simulink model "AutogiroModel"  (R2025b)
settings: Solver=FixedStepAuto  StartTime=0.0  StopTime=170  FixedStep=0.01  MaxStep=0.001  RelTol=1e-2
PreLoadFcn:
  | state = "path";
  | visual3D = true;
  | lookDistance = 500;
  | kappa = 0.1;
  | hRef = 20;
  | VRef = 30;
  | WP(:,1) = [0  0  -20]';
  | WP(:,2) = [1500  0  -20]';
  | WP(:,3) = [1500  1000 -20]';
  | WP(:,4) = [0  1000  -20]';
  | WP(:,5) = [0  0  -20]';
model workspace (MAT data in the model file):
  L1 = 3.13
undefined symbols (not defined in the file): gravity, m, rad, rho, s, WP
libraries: slpidlib x9, aerolibconvert2 x5, simulink x3, simulink_extras x3, matrix_library x2, aerolibsim3d x2, aerolibatmos2 x1, aerolibobsolete x1, aerolibasang x1, sim3dlib x1
(part 3 of 4)

== system AutogiroModel/Environment ==
  states : Inport
  Bus Creator : BusCreator  Inputs=gravity,rho
  Bus Selector : BusSelector  OutputSignals=Xe
  COESA Atmosphere Model : aerolibatmos2/COESA Atmosphere Model  units=Metric (MKS)  spec=1976 COESA-extended U.S. Standard Atmosphere  model=Profile  profile_var=High temperature  profile_percent=1%  profile_alt=5 km (16404 ft)  envelope_var=High temperature  envelope_percent=1%  action=None
  Gain : Gain  Gain=-1
  Selector : Selector  InputPortWidth=3  IndexOptions=Index vector (dialog)  Indices=[3]  OutputSizes=1
  Terminator : Terminator
  Terminator1 : Terminator
  Terminator2 : Terminator
  gravityNED : Constant  Value=[0 0 9.81]
  statesEnv : Outport
  wires:
  Gain/1 -> COESA Atmosphere Model/1
  COESA Atmosphere Model/4 -> Bus Creator/2  "rho"
  COESA Atmosphere Model/1 -> Terminator/1
  COESA Atmosphere Model/3 -> Terminator2/1
  COESA Atmosphere Model/2 -> Terminator1/1
  gravityNED/1 -> Bus Creator/1  "gravity"
  Bus Creator/1 -> statesEnv/1
  states/1 -> Bus Selector/1
  Bus Selector/1 -> Selector/1  "<Xe>"
  Selector/1 -> Gain/1

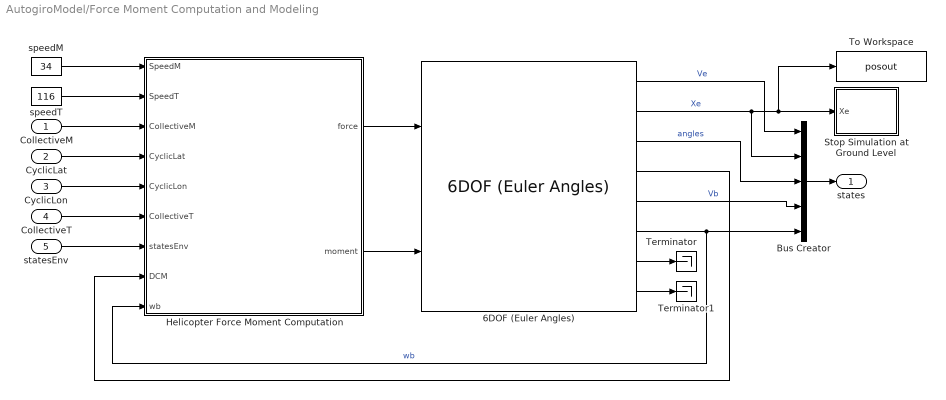
== system AutogiroModel/Force Moment Computation and Modeling ==
  CollectiveM : Inport
  CyclicLat : Inport  Port=2
  CyclicLon : Inport  Port=3
  CollectiveT : Inport  Port=4
  statesEnv : Inport  Port=5
  6DOF (Euler Angles) : aerolibobsolete/6DOF (Euler Angles)  units=Metric (MKS)  mtype=Fixed  rep=Euler Angles  xme_0=[0 0 0]  Vm_0=[0 0 0]  eul_0=[0 0 0]  pm_0=[0 0 0]  mass_0=2800  mass_e=0.5  mass_f=2.0  inertia=[3795 0 2006;0 17259 0;0 0 14639]  inertia_e=eye(3)  inertia_f=2*eye(3)  k_quat=1.0  vre_flag=on  abi_flag=off  aMode=0  xme_statename=''  Vm_statename=''  eul_statename=''  quat_statename=''  pm_statename=''  mass_statename=''
  Bus Creator : BusCreator  Inputs=5
  Helicopter Force Moment Computation : Subsystem
  Stop Simulation at Ground Level : Subsystem
  Terminator : Terminator
  Terminator1 : Terminator
  To Workspace : ToWorkspace  VariableName=posout  SaveFormat=Timeseries  SampleTime=-1
  speedM : Constant  Value=34
  speedT : Constant  Value=116
  states : Outport
  wires:
  6DOF (Euler Angles)/6 -> Bus Creator/5, Helicopter Force Moment Computation/9(wb)  "wb"
  6DOF (Euler Angles)/7 -> Terminator/1
  CyclicLat/1 -> Helicopter Force Moment Computation/4(CyclicLat)
  6DOF (Euler Angles)/5 -> Bus Creator/4  "Vb"
  6DOF (Euler Angles)/8 -> Terminator1/1
  Helicopter Force Moment Computation/1(force) -> 6DOF (Euler Angles)/1
  6DOF (Euler Angles)/2 -> To Workspace/1, Stop Simulation at Ground Level/1(Xe), Bus Creator/2  "Xe"
  6DOF (Euler Angles)/3 -> Bus Creator/3  "angles"
  CyclicLon/1 -> Helicopter Force Moment Computation/5(CyclicLon)
  CollectiveM/1 -> Helicopter Force Moment Computation/3(CollectiveM)
  CollectiveT/1 -> Helicopter Force Moment Computation/6(CollectiveT)
  Helicopter Force Moment Computation/2(moment) -> 6DOF (Euler Angles)/2
  6DOF (Euler Angles)/4 -> Helicopter Force Moment Computation/8(DCM)
  6DOF (Euler Angles)/1 -> Bus Creator/1  "Ve"
  Bus Creator/1 -> states/1
  speedM/1 -> Helicopter Force Moment Computation/1(SpeedM)
  speedT/1 -> Helicopter Force Moment Computation/2(SpeedT)
  statesEnv/1 -> Helicopter Force Moment Computation/7(statesEnv)

== system AutogiroModel/Instrument Panel ==
  Airspeed Indicator : AirspeedIndicatorBlock  LabelPosition=Hide  ScaleMin=0  ScaleMax=450
  Altimeter : AltimeterBlock  LabelPosition=Hide
  Artificial Horizon : ArtificialHorizonBlock  LabelPosition=Hide
  Climb Rate Indicator : ClimbIndicatorBlock  LabelPosition=Hide  ScaleMax=16000
  Heading Indicator : HeadingIndicatorBlock  LabelPosition=Hide
  Turn Coordinator : TurnCoordinatorBlock  LabelPosition=Hide

== system AutogiroModel/Sensor ==
  states : Inport
  Bias : Bias  Bias=0.0  SaturateOnIntegerOverflow=off
  Bus Creator : BusCreator  Inputs=5
  Bus Selector : BusSelector  OutputSignals=Ve,Xe,angles,Vb,wb
  Demux : Demux  Outputs=5
  For Each Subsystem : Subsystem  TreatAsAtomicUnit=on
  Gain : Gain  Gain=0.01
  Sum{,1..4} (5 alike) : Sum  Inputs=|++
  Uniform Random Number : UniformRandomNumber  Minimum=-0.05  Maximum=0.05  Seed=1:15  SampleTime=0.1  VectorParams1D=off
  output : Outport
  wires:
  states/1 -> Bus Selector/1
  Bus Selector/1 -> Sum/1  "<Ve>"
  Sum/1 -> Bus Creator/1  "Ve"
  Bus Creator/1 -> output/1
  Bus Selector/5 -> Sum4/1  "<wb>"
  Bus Selector/4 -> Sum3/1  "<Vb>"
  Bus Selector/3 -> Sum2/1  "<angles>"
  Bus Selector/2 -> Sum1/1  "<Xe>"
  Sum1/1 -> Bus Creator/2  "Xe"
  Sum3/1 -> Bus Creator/4  "Vb"
  Sum4/1 -> Bus Creator/5  "wb"
  Sum2/1 -> Bus Creator/3  "angles"
  Uniform Random Number/1 -> Gain/1
  Gain/1 -> Bias/1
  Bias/1 -> For Each Subsystem/1(discrete)
  Demux/1 -> Sum4/2
  Demux/2 -> Sum3/2
  Demux/3 -> Sum2/2
  Demux/4 -> Sum1/2
  Demux/5 -> Sum/2
  For Each Subsystem/1(cont) -> Demux/1

== system AutogiroModel/Visualization ==
  states : Inport
  Extract Flight Instruments : Subsystem
  Terminator{,1..5} (6 alike) : Terminator
  Variant Subsystem : Subsystem  Variant=on
  wires:
  states/1 -> Extract Flight Instruments/1(states), Variant Subsystem/1(states)
  Extract Flight Instruments/6("Turn, SlipSkid (deg)") -> Terminator5/1
  Extract Flight Instruments/5(Heading (deg)) -> Terminator4/1
  Extract Flight Instruments/4(Climb Rate (ft/min)) -> Terminator3/1
  Extract Flight Instruments/3("Roll, Pitch (deg)") -> Terminator2/1
  Extract Flight Instruments/2(Height (ft)) -> Terminator1/1
  Extract Flight Instruments/1(Airspeed (kts)) -> Terminator/1

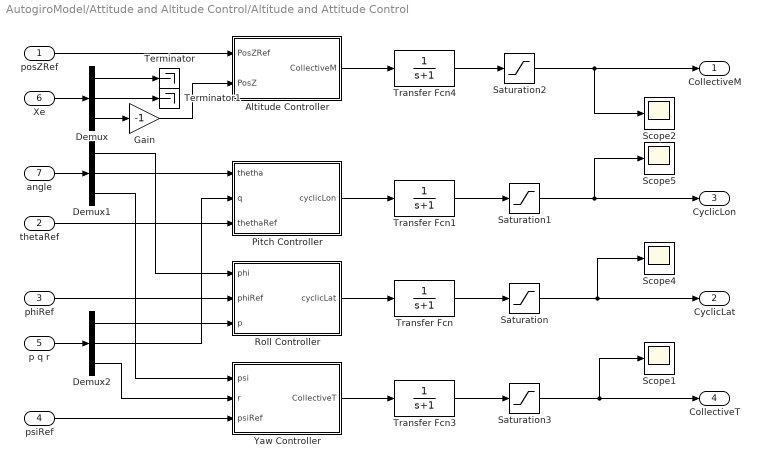
== system AutogiroModel/Attitude and Altitude Control/Altitude and Attitude Control ==
  posZRef : Inport
  thetaRef : Inport  Port=2
  phiRef : Inport  Port=3
  psiRef : Inport  Port=4
  p q r : Inport  Port=5
  Xe : Inport  Port=6
  angle : Inport  Port=7
  Altitude Controller : Subsystem
  Demux : Demux  Outputs=3
  Demux1 : Demux  Outputs=3
  Demux2 : Demux  Outputs=3
  Gain : Gain  Gain=-1
  Pitch Controller : Subsystem
  Roll Controller : Subsystem
  Saturation : Saturate  UpperLimit=0.21  LowerLimit=-0.21
  Saturation1 : Saturate  UpperLimit=0.21  LowerLimit=-0.21
  Saturation2 : Saturate  UpperLimit=0.15  LowerLimit=0.08
  Saturation3 : Saturate
  Scope{1..2,4..5} (4 alike) : Scope
      Scope1 settings: ActiveDisplayYMinimum=-0.02233  ActiveDisplayYMaximum=0.0758  DataLoggingVariableName=ScopeData3
      Scope2 settings: ActiveDisplayYMinimum=0.07554  ActiveDisplayYMaximum=0.12014
      Scope4 settings: ActiveDisplayYMinimum=-0.02233  ActiveDisplayYMaximum=0.0758
      Scope5 settings: ActiveDisplayYMinimum=-0.01721  ActiveDisplayYMaximum=0.02812  DataLoggingVariableName=ScopeData2
  Terminator : Terminator
  Terminator1 : Terminator
  Transfer Fcn{,1,3..4} (4 alike) : TransferFcn  Denominator=[1 1]
  Yaw Controller : Subsystem
  CollectiveM : Outport
  CyclicLat : Outport  Port=2
  CyclicLon : Outport  Port=3
  CollectiveT : Outport  Port=4
  wires:
  Demux/3 -> Gain/1
  Xe/1 -> Demux/1
  Demux2/1 -> Roll Controller/3(p)
  p q r/1 -> Demux2/1
  Saturation2/1 -> Scope2/1, CollectiveM/1
  Saturation3/1 -> Scope1/1, CollectiveT/1
  Saturation/1 -> Scope4/1, CyclicLat/1
  Saturation1/1 -> CyclicLon/1, Scope5/1
  Transfer Fcn1/1 -> Saturation1/1
  Transfer Fcn/1 -> Saturation/1
  Roll Controller/1(cyclicLat) -> Transfer Fcn/1
  Demux2/2 -> Pitch Controller/2(q)
  Pitch Controller/1(cyclicLon) -> Transfer Fcn1/1
  angle/1 -> Demux1/1
  Demux1/1 -> Roll Controller/1(phi)
  Demux1/2 -> Pitch Controller/1(thetha)
  Transfer Fcn4/1 -> Saturation2/1
  Altitude Controller/1(CollectiveM) -> Transfer Fcn4/1
  Transfer Fcn3/1 -> Saturation3/1
  Yaw Controller/1(CollectiveT) -> Transfer Fcn3/1
  Demux2/3 -> Yaw Controller/2(r)
  Demux1/3 -> Yaw Controller/1(psi)
  Gain/1 -> Altitude Controller/2(PosZ)
  posZRef/1 -> Altitude Controller/1(PosZRef)
  thetaRef/1 -> Pitch Controller/3(thethaRef)
  phiRef/1 -> Roll Controller/2(phiRef)
  Demux/2 -> Terminator1/1
  Demux/1 -> Terminator/1
  psiRef/1 -> Yaw Controller/3(psiRef)

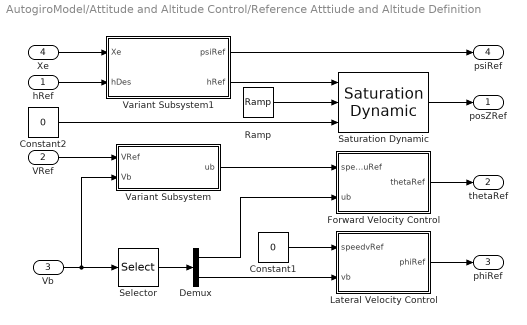
== system AutogiroModel/Attitude and Altitude Control/Reference Atttiude and Altitude Definition ==
  hRef : Inport
  VRef : Inport  Port=2
  Vb : Inport  Port=3
  Xe : Inport  Port=4
  Constant1 : Constant  Value=0
  Constant2 : Constant  Value=0
  Demux : Demux  Outputs=2
  Forward Velocity Control : Subsystem
  Lateral Velocity Control : Subsystem
  Ramp : simulink/Sources/Ramp  slope=8  start=0  InitialOutput=0
  Saturation Dynamic : simulink/Discontinuities/Saturation Dynamic  OutMin=[]  OutMax=[]  OutDataTypeStr=Inherit: Same as second input  OutDataType=fixdt(1, 16)  OutScaling=2^-10  DoSatur=off
  Selector : Selector  InputPortWidth=3  IndexOptions=Index vector (dialog)  Indices=[1 2]  OutputSizes=1
  Variant Subsystem : Subsystem  Variant=on
  Variant Subsystem1 : Subsystem  Variant=on
  posZRef : Outport
  thetaRef : Outport  Port=2
  phiRef : Outport  Port=3
  psiRef : Outport  Port=4
  wires:
  Constant1/1 -> Lateral Velocity Control/1(speedvRef)
  Vb/1 -> Selector/1, Variant Subsystem/2(Vb)
  Lateral Velocity Control/1(phiRef) -> phiRef/1
  Forward Velocity Control/1(thetaRef) -> thetaRef/1
  Ramp/1 -> Saturation Dynamic/2
  Saturation Dynamic/1 -> posZRef/1
  Variant Subsystem/1(ub) -> Forward Velocity Control/1(speeduRef)
  Selector/1 -> Demux/1
  Demux/2 -> Lateral Velocity Control/2(vb)
  Demux/1 -> Forward Velocity Control/2(ub)
  Constant2/1 -> Saturation Dynamic/3
  VRef/1 -> Variant Subsystem/1(VRef)
  Xe/1 -> Variant Subsystem1/1(Xe)
  hRef/1 -> Variant Subsystem1/2(hDes)
  Variant Subsystem1/2(hRef) -> Saturation Dynamic/1
  Variant Subsystem1/1(psiRef) -> psiRef/1

== system AutogiroModel/Force Moment Computation and Modeling/Helicopter Force Moment Computation ==
  SpeedM : Inport
  SpeedT : Inport  Port=2
  CollectiveM : Inport  Port=3
  CyclicLat : Inport  Port=4
  CyclicLon : Inport  Port=5
  CollectiveT : Inport  Port=6
  statesEnv : Inport  Port=7
  DCM : Inport  Port=8
  wb : Inport  Port=9
  ComputeForceandMoment : Subsystem
  ResultantForcesandMoments : Subsystem
  force : Outport
  moment : Outport  Port=2
  wires:
  ComputeForceandMoment/3(Ft) -> ResultantForcesandMoments/3(Ft)
  ComputeForceandMoment/4(Mt) -> ResultantForcesandMoments/4(Mt)
  ComputeForceandMoment/1(Fm) -> ResultantForcesandMoments/1(Fm)
  ComputeForceandMoment/5(Ff) -> ResultantForcesandMoments/5(Ff)
  ComputeForceandMoment/6(Mf) -> ResultantForcesandMoments/6(Mf)
  ComputeForceandMoment/7(Fg) -> ResultantForcesandMoments/7(Fg)
  ComputeForceandMoment/2(Mm) -> ResultantForcesandMoments/2(Mm)
  wb/1 -> ComputeForceandMoment/8(wb)
  ResultantForcesandMoments/2(moment) -> moment/1
  ResultantForcesandMoments/1(force) -> force/1
  SpeedM/1 -> ComputeForceandMoment/1(SpeedM)
  SpeedT/1 -> ComputeForceandMoment/2(SpeedT)
  CollectiveM/1 -> ComputeForceandMoment/3(CollectiveM)
  CollectiveT/1 -> ComputeForceandMoment/6(CollectiveT)
  ComputeForceandMoment/8(Fv) -> ResultantForcesandMoments/8(Fv)
  ComputeForceandMoment/9(Mv) -> ResultantForcesandMoments/9(Mv)
  ComputeForceandMoment/10(Fh) -> ResultantForcesandMoments/10(Fh)
  ComputeForceandMoment/11(Mh) -> ResultantForcesandMoments/11(Mh)
  statesEnv/1 -> ComputeForceandMoment/9(statesEnv)
  DCM/1 -> ComputeForceandMoment/7(DCM)
  CyclicLon/1 -> ComputeForceandMoment/4(CyclicLon)
  CyclicLat/1 -> ComputeForceandMoment/5(CyclicLat)

== system AutogiroModel/Force Moment Computation and Modeling/Stop Simulation at Ground Level ==
  Xe : Inport
  Compare To Constant : simulink/Logic and Bit Operations/Compare To Constant  relop=>  const=0.1  OutDataTypeStr=boolean
  Selector : Selector  InputPortWidth=3  IndexOptions=Index vector (dialog)  Indices=[3]  OutputSizes=1
  Stop Simulation : Stop
  wires:
  Compare To Constant/1 -> Stop Simulation/1
  Xe/1 -> Selector/1
  Selector/1 -> Compare To Constant/1

== system AutogiroModel/Sensor/For Each Subsystem ==
  discrete : Inport  Partition=on  PartitionDimension=1  PartitionWidth=1  PartitionOffset=0
  First Order Hold : FirstOrderHold  ErrorTolerance=inf
  For Each : ForEach  DisableCoverage=on
  cont : Outport  ConcatenationDimension=1
  wires:
  discrete/1 -> First Order Hold/1
  First Order Hold/1 -> cont/1

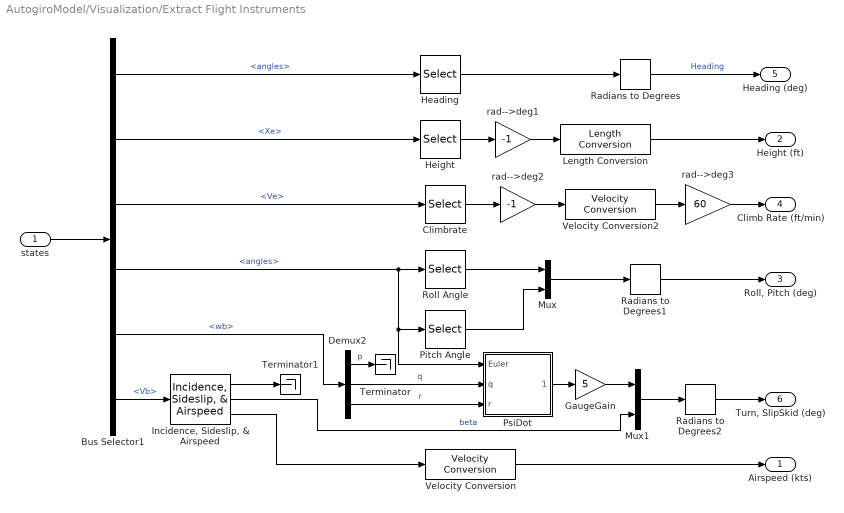
== system AutogiroModel/Visualization/Extract Flight Instruments ==
  states : Inport
  Bus Selector1 : BusSelector  OutputSignals=angles,Xe,Ve,angles,wb,Vb
  Climbrate : Selector  IndexMode=Zero-based  InputPortWidth=3  IndexOptions=Index vector (dialog)  Indices=2  OutputSizes=1
  Demux2 : Demux  Outputs=3
  GaugeGain : Gain  Gain=5
  Heading : Selector  IndexMode=Zero-based  InputPortWidth=3  IndexOptions=Index vector (dialog)  Indices=2  OutputSizes=1
  Height : Selector  IndexMode=Zero-based  InputPortWidth=3  IndexOptions=Index vector (dialog)  Indices=2  OutputSizes=1
  "Incidence, Sideslip, & Airspeed" : aerolibasang/Incidence, Sideslip, & Airspeed
  Length Conversion : aerolibconvert2/Length Conversion  IU=m  OU=ft
  Mux : Mux  Inputs=2
  Mux1 : Mux  Inputs=2
  Pitch Angle : Selector  IndexMode=Zero-based  InputPortWidth=3  IndexOptions=Index vector (dialog)  Indices=1  OutputSizes=1
  PsiDot : Subsystem
  Radians to Degrees : simulink_extras/Transformations/Radians to Degrees
  Radians to Degrees1 : simulink_extras/Transformations/Radians to Degrees
  Radians to Degrees2 : simulink_extras/Transformations/Radians to Degrees
  Roll Angle : Selector  IndexMode=Zero-based  InputPortWidth=3  IndexOptions=Index vector (dialog)  Indices=0  OutputSizes=1
  Terminator : Terminator
  Terminator1 : Terminator
  Velocity Conversion : aerolibconvert2/Velocity Conversion  IU=m/s  OU=kts
  Velocity Conversion2 : aerolibconvert2/Velocity Conversion  IU=m/s  OU=kts
  rad-->deg1 : Gain  Gain=-1  SaturateOnIntegerOverflow=on  OutDataTypeStr=Inherit: Same as input  ParamDataTypeStr=Inherit: Same as input
  rad-->deg2 : Gain  Gain=-1  SaturateOnIntegerOverflow=on  OutDataTypeStr=Inherit: Same as input  ParamDataTypeStr=Inherit: Same as input
  rad-->deg3 : Gain  Gain=60  SaturateOnIntegerOverflow=on  OutDataTypeStr=Inherit: Same as input  ParamDataTypeStr=Inherit: Same as input
  Airspeed (kts) : Outport  Unit=kn  VectorParamsAs1DForOutWhenUnconnected=off
  Height (ft) : Outport  Port=2  Unit=ft  VectorParamsAs1DForOutWhenUnconnected=off
  "Roll, Pitch (deg)" : Outport  Port=3  Unit=deg  VectorParamsAs1DForOutWhenUnconnected=off
  Climb Rate (ft/min) : Outport  Port=4  Unit=ft/min  VectorParamsAs1DForOutWhenUnconnected=off
  Heading (deg) : Outport  Port=5  Unit=deg  VectorParamsAs1DForOutWhenUnconnected=off
  "Turn, SlipSkid (deg)" : Outport  Port=6  Unit=deg  VectorParamsAs1DForOutWhenUnconnected=off
  wires:
  Radians to Degrees1/1 -> "Roll, Pitch (deg)"/1
  Mux/1 -> Radians to Degrees1/1
  Roll Angle/1 -> Mux/1
  rad-->deg3/1 -> Climb Rate (ft/min)/1
  Velocity Conversion2/1 -> rad-->deg3/1
  Bus Selector1/3 -> Climbrate/1  "<Ve>"
  rad-->deg2/1 -> Velocity Conversion2/1
  Climbrate/1 -> rad-->deg2/1
  Length Conversion/1 -> Height (ft)/1
  rad-->deg1/1 -> Length Conversion/1
  Height/1 -> rad-->deg1/1
  Bus Selector1/2 -> Height/1  "<Xe>"
  Radians to Degrees/1 -> Heading (deg)/1  "Heading"
  Heading/1 -> Radians to Degrees/1
  Bus Selector1/1 -> Heading/1  "<angles>"
  Velocity Conversion/1 -> Airspeed (kts)/1
  "Incidence, Sideslip, & Airspeed"/3 -> Velocity Conversion/1
  Pitch Angle/1 -> Mux/2
  Bus Selector1/4 -> Pitch Angle/1, PsiDot/1(Euler), Roll Angle/1  "<angles>"
  Demux2/3 -> PsiDot/3(r)  "r"
  "Incidence, Sideslip, & Airspeed"/2 -> Mux1/2  "beta"
  GaugeGain/1 -> Mux1/1
  Demux2/1 -> Terminator/1  "p"
  Demux2/2 -> PsiDot/2(q)  "q"
  Bus Selector1/5 -> Demux2/1  "<wb>"
  PsiDot/1(psi_dot) -> GaugeGain/1
  Mux1/1 -> Radians to Degrees2/1
  Radians to Degrees2/1 -> "Turn, SlipSkid (deg)"/1
  states/1 -> Bus Selector1/1
  Bus Selector1/6 -> "Incidence, Sideslip, & Airspeed"/1  "<Vb>"
  "Incidence, Sideslip, & Airspeed"/1 -> Terminator1/1

== system AutogiroModel/Visualization/Variant Subsystem ==
  note: Set visual = true to visualize using Simulink 3D Animation and
      | visual = false to visualize scope results without enabling Simulink 3D Animation
  states : Inport
  Scope Visualization : Subsystem  VariantControl=visual3D == false
  Simulink 3D Animation : Subsystem  VariantControl=visual3D == true

== system AutogiroModel/Attitude and Altitude Control/Altitude and Attitude Control/Altitude Controller ==
  PosZRef : Inport
  PosZ : Inport  Port=2
  PID Controller3 : slpidlib/PID Controller  Controller=PID  Form=Parallel  TimeDomain=Continuous-time  UseExternalTs=off  SampleTime=-1  IntegratorMethod=Forward Euler  FilterMethod=Forward Euler  ControllerParametersSource=internal  P=0.09  I=0.02  UseKiTs=off  D=1  UseExternalDerivativeSource=off  N=200  UseFilter=on  TunerSelectOption=Transfer Function Based (PID Tuner App)  InitialConditionSource=internal  InitialConditionForIntegrator=0  InitialConditionForFilter=0  DifferentiatorICPrevScaledInput=0  ExternalReset=none  TrackingMode=off  Kt=10  LimitOutput=on  SatLimitsSource=internal  UpperSaturationLimit=0.2  LowerSaturationLimit=0  LinearizeAsGain=on  AntiWindupMode=back-calculation  Kb=10  LimitIntegrator=off  UpperIntegratorSaturationLimit=inf  LowerIntegratorSaturationLimit=-inf  POutMin=[]  POutMax=[]  IOutMin=[]  IOutMax=[]  DOutMin=[]  DOutMax=[]  NOutMin=[]  NOutMax=[]  SumOutMin=[]  SumOutMax=[]  SaturationOutMin=[]  SaturationOutMax=[]  PParamMin=[]  PParamMax=[]  IParamMin=[]  IParamMax=[]  DParamMin=[]  DParamMax=[]  NParamMin=[]  NParamMax=[]  KbParamMin=[]  KbParamMax=[]  KtParamMin=[]  KtParamMax=[]  KbOutMin=[]  KbOutMax=[]  KtOutMin=[]  KtOutMax=[]  IntegratorOutMin=[]  IntegratorOutMax=[]  FilterOutMin=[]  FilterOutMax=[]  SumI1OutMin=[]  SumI1OutMax=[]  SumI2OutMin=[]  SumI2OutMax=[]  SumI3OutMin=[]  SumI3OutMax=[]  SumI4OutMin=[]  SumI4OutMax=[]  SumDOutMin=[]  SumDOutMax=[]  DifferentiatorOutMin=[]  DifferentiatorOutMax=[]  FilterDiffOutCoefMin=[]  FilterDiffOutCoefMax=[]  ReciprocalOutMin=[]  ReciprocalOutMax=[]  SumDenOutMin=[]  SumDenOutMax=[]  SumNumOutMin=[]  SumNumOutMax=[]  DivideOutMin=[]  DivideOutMax=[]  UdiffTsProdOutMin=[]  UdiffTsProdOutMax=[]  NTsProdOutMin=[]  NTsProdOutMax=[]  UintegralTsProdOutMin=[]  UintegralTsProdOutMax=[]  UngainTsProdOutMin=[]  UngainTsProdOutMax=[]  ClampingZeroOutDataTypeStr=Inherit: Inherit via back propagation  ClampingZeroOutMin=[]  ClampingZeroOutMax=[]  FilterDenConstantOutDataTypeStr=Inherit: Inherit via back propagation  FilterDenConstantOutMin=[]  FilterDenConstantOutMax=[]  PCopyOutDataTypeStr=Inherit: Inherit via back propagation  PCopyOutMin=[]  PCopyOutMax=[]  NCopyOutDataTypeStr=Inherit: Inherit via back propagation  NCopyOutMin=[]  NCopyOutMax=[]  IntegratorContinuousStateAttributes=''  IntegratorStateMustResolveToSignalObject=off  IntegratorRTWStateStorageClass=Auto  FilterContinuousStateAttributes=''  FilterStateMustResolveToSignalObject=off  FilterRTWStateStorageClass=Auto  ParallelPVariant=InternalParameters  IdealPVariant=Disabled  IVariant=InternalParameters  DVariant=InternalParameters  IntegratorVariant=Continuous  SatVariant=Enabled  AWVariant=BackCalculation  PCopyVariant=Disabled  TRVariant=Disabled  FdbkBlocksVariant=Forward  IdealPFdbkVariant=Disabled  SatFdbkVariant=Disabled  DerivativeFilterVariant=ContFilter  NVariant=InternalParameters  NCopyVariant=Disabled  FilterICVariant=InternalICsFilter  IntegratorICVariant=InternalICs  ExternalResetVariant=Disabled  TRSumVariant=Passthrough  SumFdbkVariant=Disabled  SumVariant=Sum_PID  TsampFilterVariant=InternalTs  TsampNgainVariant=Passthrough  TsampIntegralVariant=Disabled_SignalSpec  ExternalSaturationOutDataTypeStr=Inherit: Same as second input  DerivativeSourceVariant=ErrorSignal  PreIntVariant=InternalPreInt
  Sum : Sum  Inputs=|+-
  CollectiveM : Outport  VectorParamsAs1DForOutWhenUnconnected=off
  wires:
  PosZ/1 -> Sum/2
  PosZRef/1 -> Sum/1
  Sum/1 -> PID Controller3/1
  PID Controller3/1 -> CollectiveM/1

== system AutogiroModel/Attitude and Altitude Control/Altitude and Attitude Control/Pitch Controller ==
  thetha : Inport
  q : Inport  Port=2
  thethaRef : Inport  Port=3
  PID Controller : slpidlib/PID Controller  Controller=PID  Form=Parallel  TimeDomain=Continuous-time  UseExternalTs=off  SampleTime=-1  IntegratorMethod=Forward Euler  FilterMethod=Forward Euler  ControllerParametersSource=internal  P=2  I=0.01  UseKiTs=off  D=0  UseExternalDerivativeSource=off  N=50  UseFilter=on  TunerSelectOption=Transfer Function Based (PID Tuner App)  InitialConditionSource=internal  InitialConditionForIntegrator=0  InitialConditionForFilter=0  DifferentiatorICPrevScaledInput=0  ExternalReset=none  TrackingMode=off  Kt=10  LimitOutput=on  SatLimitsSource=internal  UpperSaturationLimit=0.21  LowerSaturationLimit=-0.21  LinearizeAsGain=on  AntiWindupMode=back-calculation  Kb=1  LimitIntegrator=off  UpperIntegratorSaturationLimit=inf  LowerIntegratorSaturationLimit=-inf  POutMin=[]  POutMax=[]  IOutMin=[]  IOutMax=[]  DOutMin=[]  DOutMax=[]  NOutMin=[]  NOutMax=[]  SumOutMin=[]  SumOutMax=[]  SaturationOutMin=[]  SaturationOutMax=[]  PParamMin=[]  PParamMax=[]  IParamMin=[]  IParamMax=[]  DParamMin=[]  DParamMax=[]  NParamMin=[]  NParamMax=[]  KbParamMin=[]  KbParamMax=[]  KtParamMin=[]  KtParamMax=[]  KbOutMin=[]  KbOutMax=[]  KtOutMin=[]  KtOutMax=[]  IntegratorOutMin=[]  IntegratorOutMax=[]  FilterOutMin=[]  FilterOutMax=[]  SumI1OutMin=[]  SumI1OutMax=[]  SumI2OutMin=[]  SumI2OutMax=[]  SumI3OutMin=[]  SumI3OutMax=[]  SumI4OutMin=[]  SumI4OutMax=[]  SumDOutMin=[]  SumDOutMax=[]  DifferentiatorOutMin=[]  DifferentiatorOutMax=[]  FilterDiffOutCoefMin=[]  FilterDiffOutCoefMax=[]  ReciprocalOutMin=[]  ReciprocalOutMax=[]  SumDenOutMin=[]  SumDenOutMax=[]  SumNumOutMin=[]  SumNumOutMax=[]  DivideOutMin=[]  DivideOutMax=[]  UdiffTsProdOutMin=[]  UdiffTsProdOutMax=[]  NTsProdOutMin=[]  NTsProdOutMax=[]  UintegralTsProdOutMin=[]  UintegralTsProdOutMax=[]  UngainTsProdOutMin=[]  UngainTsProdOutMax=[]  ClampingZeroOutDataTypeStr=Inherit: Inherit via back propagation  ClampingZeroOutMin=[]  ClampingZeroOutMax=[]  FilterDenConstantOutDataTypeStr=Inherit: Inherit via back propagation  FilterDenConstantOutMin=[]  FilterDenConstantOutMax=[]  PCopyOutDataTypeStr=Inherit: Inherit via back propagation  PCopyOutMin=[]  PCopyOutMax=[]  NCopyOutDataTypeStr=Inherit: Inherit via back propagation  NCopyOutMin=[]  NCopyOutMax=[]  IntegratorContinuousStateAttributes=''  IntegratorStateMustResolveToSignalObject=off  IntegratorRTWStateStorageClass=Auto  FilterContinuousStateAttributes=''  FilterStateMustResolveToSignalObject=off  FilterRTWStateStorageClass=Auto  ParallelPVariant=InternalParameters  IdealPVariant=Disabled  IVariant=InternalParameters  DVariant=InternalParameters  IntegratorVariant=Continuous  SatVariant=Enabled  AWVariant=BackCalculation  PCopyVariant=Disabled  TRVariant=Disabled  FdbkBlocksVariant=Forward  IdealPFdbkVariant=Disabled  SatFdbkVariant=Disabled  DerivativeFilterVariant=ContFilter  NVariant=InternalParameters  NCopyVariant=Disabled  FilterICVariant=InternalICsFilter  IntegratorICVariant=InternalICs  ExternalResetVariant=Disabled  TRSumVariant=Passthrough  SumFdbkVariant=Disabled  SumVariant=Sum_PID  TsampFilterVariant=InternalTs  TsampNgainVariant=Passthrough  TsampIntegralVariant=Disabled_SignalSpec  ExternalSaturationOutDataTypeStr=Inherit: Same as second input  DerivativeSourceVariant=ErrorSignal  PreIntVariant=InternalPreInt
  PID Controller2 : slpidlib/PID Controller  Controller=PID  Form=Parallel  TimeDomain=Continuous-time  UseExternalTs=off  SampleTime=-1  IntegratorMethod=Forward Euler  FilterMethod=Forward Euler  ControllerParametersSource=internal  P=0.3  I=0.05  UseKiTs=off  D=0.15  UseExternalDerivativeSource=off  N=100  UseFilter=on  TunerSelectOption=Transfer Function Based (PID Tuner App)  InitialConditionSource=internal  InitialConditionForIntegrator=0  InitialConditionForFilter=0  DifferentiatorICPrevScaledInput=0  ExternalReset=none  TrackingMode=off  Kt=10  LimitOutput=on  SatLimitsSource=internal  UpperSaturationLimit=0.35  LowerSaturationLimit=-0.35  LinearizeAsGain=on  AntiWindupMode=back-calculation  Kb=1  LimitIntegrator=off  UpperIntegratorSaturationLimit=inf  LowerIntegratorSaturationLimit=-inf  POutMin=[]  POutMax=[]  IOutMin=[]  IOutMax=[]  DOutMin=[]  DOutMax=[]  NOutMin=[]  NOutMax=[]  SumOutMin=[]  SumOutMax=[]  SaturationOutMin=[]  SaturationOutMax=[]  PParamMin=[]  PParamMax=[]  IParamMin=[]  IParamMax=[]  DParamMin=[]  DParamMax=[]  NParamMin=[]  NParamMax=[]  KbParamMin=[]  KbParamMax=[]  KtParamMin=[]  KtParamMax=[]  KbOutMin=[]  KbOutMax=[]  KtOutMin=[]  KtOutMax=[]  IntegratorOutMin=[]  IntegratorOutMax=[]  FilterOutMin=[]  FilterOutMax=[]  SumI1OutMin=[]  SumI1OutMax=[]  SumI2OutMin=[]  SumI2OutMax=[]  SumI3OutMin=[]  SumI3OutMax=[]  SumI4OutMin=[]  SumI4OutMax=[]  SumDOutMin=[]  SumDOutMax=[]  DifferentiatorOutMin=[]  DifferentiatorOutMax=[]  FilterDiffOutCoefMin=[]  FilterDiffOutCoefMax=[]  ReciprocalOutMin=[]  ReciprocalOutMax=[]  SumDenOutMin=[]  SumDenOutMax=[]  SumNumOutMin=[]  SumNumOutMax=[]  DivideOutMin=[]  DivideOutMax=[]  UdiffTsProdOutMin=[]  UdiffTsProdOutMax=[]  NTsProdOutMin=[]  NTsProdOutMax=[]  UintegralTsProdOutMin=[]  UintegralTsProdOutMax=[]  UngainTsProdOutMin=[]  UngainTsProdOutMax=[]  ClampingZeroOutDataTypeStr=Inherit: Inherit via back propagation  ClampingZeroOutMin=[]  ClampingZeroOutMax=[]  FilterDenConstantOutDataTypeStr=Inherit: Inherit via back propagation  FilterDenConstantOutMin=[]  FilterDenConstantOutMax=[]  PCopyOutDataTypeStr=Inherit: Inherit via back propagation  PCopyOutMin=[]  PCopyOutMax=[]  NCopyOutDataTypeStr=Inherit: Inherit via back propagation  NCopyOutMin=[]  NCopyOutMax=[]  IntegratorContinuousStateAttributes=''  IntegratorStateMustResolveToSignalObject=off  IntegratorRTWStateStorageClass=Auto  FilterContinuousStateAttributes=''  FilterStateMustResolveToSignalObject=off  FilterRTWStateStorageClass=Auto  ParallelPVariant=InternalParameters  IdealPVariant=Disabled  IVariant=InternalParameters  DVariant=InternalParameters  IntegratorVariant=Continuous  SatVariant=Enabled  AWVariant=BackCalculation  PCopyVariant=Disabled  TRVariant=Disabled  FdbkBlocksVariant=Forward  IdealPFdbkVariant=Disabled  SatFdbkVariant=Disabled  DerivativeFilterVariant=ContFilter  NVariant=InternalParameters  NCopyVariant=Disabled  FilterICVariant=InternalICsFilter  IntegratorICVariant=InternalICs  ExternalResetVariant=Disabled  TRSumVariant=Passthrough  SumFdbkVariant=Disabled  SumVariant=Sum_PID  TsampFilterVariant=InternalTs  TsampNgainVariant=Passthrough  TsampIntegralVariant=Disabled_SignalSpec  ExternalSaturationOutDataTypeStr=Inherit: Same as second input  DerivativeSourceVariant=ErrorSignal  PreIntVariant=InternalPreInt
  Sum1 : Sum  Inputs=|+-
  Sum2 : Sum  Inputs=|-+
  cyclicLon : Outport  VectorParamsAs1DForOutWhenUnconnected=off
  wires:
  PID Controller/1 -> cyclicLon/1
  Sum2/1 -> PID Controller/1
  q/1 -> Sum2/2
  Sum1/1 -> PID Controller2/1
  thetha/1 -> Sum1/2
  thethaRef/1 -> Sum1/1
  PID Controller2/1 -> Sum2/1

== system AutogiroModel/Attitude and Altitude Control/Altitude and Attitude Control/Roll Controller ==
  phi : Inport
  phiRef : Inport  Port=2
  p : Inport  Port=3
  PID Controller : slpidlib/PID Controller  Controller=PID  Form=Parallel  TimeDomain=Continuous-time  UseExternalTs=off  SampleTime=-1  IntegratorMethod=Forward Euler  FilterMethod=Forward Euler  ControllerParametersSource=internal  P=2  I=0.01  UseKiTs=off  D=0  UseExternalDerivativeSource=off  N=50  UseFilter=on  TunerSelectOption=Transfer Function Based (PID Tuner App)  InitialConditionSource=internal  InitialConditionForIntegrator=0  InitialConditionForFilter=0  DifferentiatorICPrevScaledInput=0  ExternalReset=none  TrackingMode=off  Kt=10  LimitOutput=on  SatLimitsSource=internal  UpperSaturationLimit=0.2  LowerSaturationLimit=-0.2  LinearizeAsGain=on  AntiWindupMode=back-calculation  Kb=1  LimitIntegrator=off  UpperIntegratorSaturationLimit=inf  LowerIntegratorSaturationLimit=-inf  POutMin=[]  POutMax=[]  IOutMin=[]  IOutMax=[]  DOutMin=[]  DOutMax=[]  NOutMin=[]  NOutMax=[]  SumOutMin=[]  SumOutMax=[]  SaturationOutMin=[]  SaturationOutMax=[]  PParamMin=[]  PParamMax=[]  IParamMin=[]  IParamMax=[]  DParamMin=[]  DParamMax=[]  NParamMin=[]  NParamMax=[]  KbParamMin=[]  KbParamMax=[]  KtParamMin=[]  KtParamMax=[]  KbOutMin=[]  KbOutMax=[]  KtOutMin=[]  KtOutMax=[]  IntegratorOutMin=[]  IntegratorOutMax=[]  FilterOutMin=[]  FilterOutMax=[]  SumI1OutMin=[]  SumI1OutMax=[]  SumI2OutMin=[]  SumI2OutMax=[]  SumI3OutMin=[]  SumI3OutMax=[]  SumI4OutMin=[]  SumI4OutMax=[]  SumDOutMin=[]  SumDOutMax=[]  DifferentiatorOutMin=[]  DifferentiatorOutMax=[]  FilterDiffOutCoefMin=[]  FilterDiffOutCoefMax=[]  ReciprocalOutMin=[]  ReciprocalOutMax=[]  SumDenOutMin=[]  SumDenOutMax=[]  SumNumOutMin=[]  SumNumOutMax=[]  DivideOutMin=[]  DivideOutMax=[]  UdiffTsProdOutMin=[]  UdiffTsProdOutMax=[]  NTsProdOutMin=[]  NTsProdOutMax=[]  UintegralTsProdOutMin=[]  UintegralTsProdOutMax=[]  UngainTsProdOutMin=[]  UngainTsProdOutMax=[]  ClampingZeroOutDataTypeStr=Inherit: Inherit via back propagation  ClampingZeroOutMin=[]  ClampingZeroOutMax=[]  FilterDenConstantOutDataTypeStr=Inherit: Inherit via back propagation  FilterDenConstantOutMin=[]  FilterDenConstantOutMax=[]  PCopyOutDataTypeStr=Inherit: Inherit via back propagation  PCopyOutMin=[]  PCopyOutMax=[]  NCopyOutDataTypeStr=Inherit: Inherit via back propagation  NCopyOutMin=[]  NCopyOutMax=[]  IntegratorContinuousStateAttributes=''  IntegratorStateMustResolveToSignalObject=off  IntegratorRTWStateStorageClass=Auto  FilterContinuousStateAttributes=''  FilterStateMustResolveToSignalObject=off  FilterRTWStateStorageClass=Auto  ParallelPVariant=InternalParameters  IdealPVariant=Disabled  IVariant=InternalParameters  DVariant=InternalParameters  IntegratorVariant=Continuous  SatVariant=Enabled  AWVariant=BackCalculation  PCopyVariant=Disabled  TRVariant=Disabled  FdbkBlocksVariant=Forward  IdealPFdbkVariant=Disabled  SatFdbkVariant=Disabled  DerivativeFilterVariant=ContFilter  NVariant=InternalParameters  NCopyVariant=Disabled  FilterICVariant=InternalICsFilter  IntegratorICVariant=InternalICs  ExternalResetVariant=Disabled  TRSumVariant=Passthrough  SumFdbkVariant=Disabled  SumVariant=Sum_PID  TsampFilterVariant=InternalTs  TsampNgainVariant=Passthrough  TsampIntegralVariant=Disabled_SignalSpec  ExternalSaturationOutDataTypeStr=Inherit: Same as second input  DerivativeSourceVariant=ErrorSignal  PreIntVariant=InternalPreInt
  PID Controller1 : slpidlib/PID Controller  Controller=PID  Form=Parallel  TimeDomain=Continuous-time  UseExternalTs=off  SampleTime=-1  IntegratorMethod=Forward Euler  FilterMethod=Forward Euler  ControllerParametersSource=internal  P=0.2  I=0.01  UseKiTs=off  D=0  UseExternalDerivativeSource=off  N=50  UseFilter=on  TunerSelectOption=Transfer Function Based (PID Tuner App)  InitialConditionSource=internal  InitialConditionForIntegrator=0  InitialConditionForFilter=0  DifferentiatorICPrevScaledInput=0  ExternalReset=none  TrackingMode=off  Kt=10  LimitOutput=on  SatLimitsSource=internal  UpperSaturationLimit=0.35  LowerSaturationLimit=-0.35  LinearizeAsGain=on  AntiWindupMode=back-calculation  Kb=1  LimitIntegrator=off  UpperIntegratorSaturationLimit=inf  LowerIntegratorSaturationLimit=-inf  POutMin=[]  POutMax=[]  IOutMin=[]  IOutMax=[]  DOutMin=[]  DOutMax=[]  NOutMin=[]  NOutMax=[]  SumOutMin=[]  SumOutMax=[]  SaturationOutMin=[]  SaturationOutMax=[]  PParamMin=[]  PParamMax=[]  IParamMin=[]  IParamMax=[]  DParamMin=[]  DParamMax=[]  NParamMin=[]  NParamMax=[]  KbParamMin=[]  KbParamMax=[]  KtParamMin=[]  KtParamMax=[]  KbOutMin=[]  KbOutMax=[]  KtOutMin=[]  KtOutMax=[]  IntegratorOutMin=[]  IntegratorOutMax=[]  FilterOutMin=[]  FilterOutMax=[]  SumI1OutMin=[]  SumI1OutMax=[]  SumI2OutMin=[]  SumI2OutMax=[]  SumI3OutMin=[]  SumI3OutMax=[]  SumI4OutMin=[]  SumI4OutMax=[]  SumDOutMin=[]  SumDOutMax=[]  DifferentiatorOutMin=[]  DifferentiatorOutMax=[]  FilterDiffOutCoefMin=[]  FilterDiffOutCoefMax=[]  ReciprocalOutMin=[]  ReciprocalOutMax=[]  SumDenOutMin=[]  SumDenOutMax=[]  SumNumOutMin=[]  SumNumOutMax=[]  DivideOutMin=[]  DivideOutMax=[]  UdiffTsProdOutMin=[]  UdiffTsProdOutMax=[]  NTsProdOutMin=[]  NTsProdOutMax=[]  UintegralTsProdOutMin=[]  UintegralTsProdOutMax=[]  UngainTsProdOutMin=[]  UngainTsProdOutMax=[]  ClampingZeroOutDataTypeStr=Inherit: Inherit via back propagation  ClampingZeroOutMin=[]  ClampingZeroOutMax=[]  FilterDenConstantOutDataTypeStr=Inherit: Inherit via back propagation  FilterDenConstantOutMin=[]  FilterDenConstantOutMax=[]  PCopyOutDataTypeStr=Inherit: Inherit via back propagation  PCopyOutMin=[]  PCopyOutMax=[]  NCopyOutDataTypeStr=Inherit: Inherit via back propagation  NCopyOutMin=[]  NCopyOutMax=[]  IntegratorContinuousStateAttributes=''  IntegratorStateMustResolveToSignalObject=off  IntegratorRTWStateStorageClass=Auto  FilterContinuousStateAttributes=''  FilterStateMustResolveToSignalObject=off  FilterRTWStateStorageClass=Auto  ParallelPVariant=InternalParameters  IdealPVariant=Disabled  IVariant=InternalParameters  DVariant=InternalParameters  IntegratorVariant=Continuous  SatVariant=Enabled  AWVariant=BackCalculation  PCopyVariant=Disabled  TRVariant=Disabled  FdbkBlocksVariant=Forward  IdealPFdbkVariant=Disabled  SatFdbkVariant=Disabled  DerivativeFilterVariant=ContFilter  NVariant=InternalParameters  NCopyVariant=Disabled  FilterICVariant=InternalICsFilter  IntegratorICVariant=InternalICs  ExternalResetVariant=Disabled  TRSumVariant=Passthrough  SumFdbkVariant=Disabled  SumVariant=Sum_PID  TsampFilterVariant=InternalTs  TsampNgainVariant=Passthrough  TsampIntegralVariant=Disabled_SignalSpec  ExternalSaturationOutDataTypeStr=Inherit: Same as second input  DerivativeSourceVariant=ErrorSignal  PreIntVariant=InternalPreInt
  Sum1 : Sum  Inputs=|+-
  Sum2 : Sum  Inputs=|+-
  cyclicLat : Outport  VectorParamsAs1DForOutWhenUnconnected=off
  wires:
  PID Controller/1 -> cyclicLat/1
  Sum2/1 -> PID Controller/1
  p/1 -> Sum2/2
  phi/1 -> Sum1/2
  phiRef/1 -> Sum1/1
  Sum1/1 -> PID Controller1/1
  PID Controller1/1 -> Sum2/1

== system AutogiroModel/Attitude and Altitude Control/Altitude and Attitude Control/Yaw Controller ==
  psi : Inport
  r : Inport  Port=2
  psiRef : Inport  Port=3
  PID Controller1 : slpidlib/PID Controller  Controller=PID  Form=Parallel  TimeDomain=Continuous-time  UseExternalTs=off  SampleTime=-1  IntegratorMethod=Forward Euler  FilterMethod=Forward Euler  ControllerParametersSource=internal  P=0.8  I=0.2  UseKiTs=off  D=0.2  UseExternalDerivativeSource=off  N=50  UseFilter=on  TunerSelectOption=Transfer Function Based (PID Tuner App)  InitialConditionSource=internal  InitialConditionForIntegrator=0  InitialConditionForFilter=0  DifferentiatorICPrevScaledInput=0  ExternalReset=none  TrackingMode=off  Kt=10  LimitOutput=on  SatLimitsSource=internal  UpperSaturationLimit=0.5  LowerSaturationLimit=0  LinearizeAsGain=on  AntiWindupMode=back-calculation  Kb=1  LimitIntegrator=off  UpperIntegratorSaturationLimit=inf  LowerIntegratorSaturationLimit=-inf  POutMin=[]  POutMax=[]  IOutMin=[]  IOutMax=[]  DOutMin=[]  DOutMax=[]  NOutMin=[]  NOutMax=[]  SumOutMin=[]  SumOutMax=[]  SaturationOutMin=[]  SaturationOutMax=[]  PParamMin=[]  PParamMax=[]  IParamMin=[]  IParamMax=[]  DParamMin=[]  DParamMax=[]  NParamMin=[]  NParamMax=[]  KbParamMin=[]  KbParamMax=[]  KtParamMin=[]  KtParamMax=[]  KbOutMin=[]  KbOutMax=[]  KtOutMin=[]  KtOutMax=[]  IntegratorOutMin=[]  IntegratorOutMax=[]  FilterOutMin=[]  FilterOutMax=[]  SumI1OutMin=[]  SumI1OutMax=[]  SumI2OutMin=[]  SumI2OutMax=[]  SumI3OutMin=[]  SumI3OutMax=[]  SumI4OutMin=[]  SumI4OutMax=[]  SumDOutMin=[]  SumDOutMax=[]  DifferentiatorOutMin=[]  DifferentiatorOutMax=[]  FilterDiffOutCoefMin=[]  FilterDiffOutCoefMax=[]  ReciprocalOutMin=[]  ReciprocalOutMax=[]  SumDenOutMin=[]  SumDenOutMax=[]  SumNumOutMin=[]  SumNumOutMax=[]  DivideOutMin=[]  DivideOutMax=[]  UdiffTsProdOutMin=[]  UdiffTsProdOutMax=[]  NTsProdOutMin=[]  NTsProdOutMax=[]  UintegralTsProdOutMin=[]  UintegralTsProdOutMax=[]  UngainTsProdOutMin=[]  UngainTsProdOutMax=[]  ClampingZeroOutDataTypeStr=Inherit: Inherit via back propagation  ClampingZeroOutMin=[]  ClampingZeroOutMax=[]  FilterDenConstantOutDataTypeStr=Inherit: Inherit via back propagation  FilterDenConstantOutMin=[]  FilterDenConstantOutMax=[]  PCopyOutDataTypeStr=Inherit: Inherit via back propagation  PCopyOutMin=[]  PCopyOutMax=[]  NCopyOutDataTypeStr=Inherit: Inherit via back propagation  NCopyOutMin=[]  NCopyOutMax=[]  IntegratorContinuousStateAttributes=''  IntegratorStateMustResolveToSignalObject=off  IntegratorRTWStateStorageClass=Auto  FilterContinuousStateAttributes=''  FilterStateMustResolveToSignalObject=off  FilterRTWStateStorageClass=Auto  ParallelPVariant=InternalParameters  IdealPVariant=Disabled  IVariant=InternalParameters  DVariant=InternalParameters  IntegratorVariant=Continuous  SatVariant=Enabled  AWVariant=BackCalculation  PCopyVariant=Disabled  TRVariant=Disabled  FdbkBlocksVariant=Forward  IdealPFdbkVariant=Disabled  SatFdbkVariant=Disabled  DerivativeFilterVariant=ContFilter  NVariant=InternalParameters  NCopyVariant=Disabled  FilterICVariant=InternalICsFilter  IntegratorICVariant=InternalICs  ExternalResetVariant=Disabled  TRSumVariant=Passthrough  SumFdbkVariant=Disabled  SumVariant=Sum_PID  TsampFilterVariant=InternalTs  TsampNgainVariant=Passthrough  TsampIntegralVariant=Disabled_SignalSpec  ExternalSaturationOutDataTypeStr=Inherit: Same as second input  DerivativeSourceVariant=ErrorSignal  PreIntVariant=InternalPreInt
  PID Controller2 : slpidlib/PID Controller  Controller=PID  Form=Parallel  TimeDomain=Continuous-time  UseExternalTs=off  SampleTime=-1  IntegratorMethod=Forward Euler  FilterMethod=Forward Euler  ControllerParametersSource=internal  P=0.6  I=0.2  UseKiTs=off  D=0.15  UseExternalDerivativeSource=off  N=100  UseFilter=on  TunerSelectOption=Transfer Function Based (PID Tuner App)  InitialConditionSource=internal  InitialConditionForIntegrator=0  InitialConditionForFilter=0  DifferentiatorICPrevScaledInput=0  ExternalReset=none  TrackingMode=off  Kt=10  LimitOutput=on  SatLimitsSource=internal  UpperSaturationLimit=3.14  LowerSaturationLimit=-3.14  LinearizeAsGain=on  AntiWindupMode=back-calculation  Kb=1  LimitIntegrator=off  UpperIntegratorSaturationLimit=inf  LowerIntegratorSaturationLimit=-inf  POutMin=[]  POutMax=[]  IOutMin=[]  IOutMax=[]  DOutMin=[]  DOutMax=[]  NOutMin=[]  NOutMax=[]  SumOutMin=[]  SumOutMax=[]  SaturationOutMin=[]  SaturationOutMax=[]  PParamMin=[]  PParamMax=[]  IParamMin=[]  IParamMax=[]  DParamMin=[]  DParamMax=[]  NParamMin=[]  NParamMax=[]  KbParamMin=[]  KbParamMax=[]  KtParamMin=[]  KtParamMax=[]  KbOutMin=[]  KbOutMax=[]  KtOutMin=[]  KtOutMax=[]  IntegratorOutMin=[]  IntegratorOutMax=[]  FilterOutMin=[]  FilterOutMax=[]  SumI1OutMin=[]  SumI1OutMax=[]  SumI2OutMin=[]  SumI2OutMax=[]  SumI3OutMin=[]  SumI3OutMax=[]  SumI4OutMin=[]  SumI4OutMax=[]  SumDOutMin=[]  SumDOutMax=[]  DifferentiatorOutMin=[]  DifferentiatorOutMax=[]  FilterDiffOutCoefMin=[]  FilterDiffOutCoefMax=[]  ReciprocalOutMin=[]  ReciprocalOutMax=[]  SumDenOutMin=[]  SumDenOutMax=[]  SumNumOutMin=[]  SumNumOutMax=[]  DivideOutMin=[]  DivideOutMax=[]  UdiffTsProdOutMin=[]  UdiffTsProdOutMax=[]  NTsProdOutMin=[]  NTsProdOutMax=[]  UintegralTsProdOutMin=[]  UintegralTsProdOutMax=[]  UngainTsProdOutMin=[]  UngainTsProdOutMax=[]  ClampingZeroOutDataTypeStr=Inherit: Inherit via back propagation  ClampingZeroOutMin=[]  ClampingZeroOutMax=[]  FilterDenConstantOutDataTypeStr=Inherit: Inherit via back propagation  FilterDenConstantOutMin=[]  FilterDenConstantOutMax=[]  PCopyOutDataTypeStr=Inherit: Inherit via back propagation  PCopyOutMin=[]  PCopyOutMax=[]  NCopyOutDataTypeStr=Inherit: Inherit via back propagation  NCopyOutMin=[]  NCopyOutMax=[]  IntegratorContinuousStateAttributes=''  IntegratorStateMustResolveToSignalObject=off  IntegratorRTWStateStorageClass=Auto  FilterContinuousStateAttributes=''  FilterStateMustResolveToSignalObject=off  FilterRTWStateStorageClass=Auto  ParallelPVariant=InternalParameters  IdealPVariant=Disabled  IVariant=InternalParameters  DVariant=InternalParameters  IntegratorVariant=Continuous  SatVariant=Enabled  AWVariant=BackCalculation  PCopyVariant=Disabled  TRVariant=Disabled  FdbkBlocksVariant=Forward  IdealPFdbkVariant=Disabled  SatFdbkVariant=Disabled  DerivativeFilterVariant=ContFilter  NVariant=InternalParameters  NCopyVariant=Disabled  FilterICVariant=InternalICsFilter  IntegratorICVariant=InternalICs  ExternalResetVariant=Disabled  TRSumVariant=Passthrough  SumFdbkVariant=Disabled  SumVariant=Sum_PID  TsampFilterVariant=InternalTs  TsampNgainVariant=Passthrough  TsampIntegralVariant=Disabled_SignalSpec  ExternalSaturationOutDataTypeStr=Inherit: Same as second input  DerivativeSourceVariant=ErrorSignal  PreIntVariant=InternalPreInt
  Sum1 : Sum  Inputs=|+-
  Sum2 : Sum  Inputs=|+-
  CollectiveT : Outport  VectorParamsAs1DForOutWhenUnconnected=off
  wires:
  PID Controller1/1 -> CollectiveT/1
  Sum2/1 -> PID Controller1/1
  r/1 -> Sum2/2
  PID Controller2/1 -> Sum2/1
  psiRef/1 -> Sum1/1
  psi/1 -> Sum1/2
  Sum1/1 -> PID Controller2/1

== system AutogiroModel/Attitude and Altitude Control/Reference Atttiude and Altitude Definition/Forward Velocity Control ==
  speeduRef : Inport
  ub : Inport  Port=2
  PID Controller1 : slpidlib/PID Controller  Controller=PID  Form=Parallel  TimeDomain=Continuous-time  UseExternalTs=off  SampleTime=-1  IntegratorMethod=Forward Euler  FilterMethod=Forward Euler  ControllerParametersSource=internal  P=0.05  I=0.01  UseKiTs=off  D=0.1  UseExternalDerivativeSource=off  N=100  UseFilter=on  TunerSelectOption=Transfer Function Based (PID Tuner App)  InitialConditionSource=internal  InitialConditionForIntegrator=0  InitialConditionForFilter=0  DifferentiatorICPrevScaledInput=0  ExternalReset=none  TrackingMode=off  Kt=10  LimitOutput=on  SatLimitsSource=internal  UpperSaturationLimit=0.35  LowerSaturationLimit=-0.35  LinearizeAsGain=on  AntiWindupMode=back-calculation  Kb=5  LimitIntegrator=off  UpperIntegratorSaturationLimit=inf  LowerIntegratorSaturationLimit=-inf  POutMin=[]  POutMax=[]  IOutMin=[]  IOutMax=[]  DOutMin=[]  DOutMax=[]  NOutMin=[]  NOutMax=[]  SumOutMin=[]  SumOutMax=[]  SaturationOutMin=[]  SaturationOutMax=[]  PParamMin=[]  PParamMax=[]  IParamMin=[]  IParamMax=[]  DParamMin=[]  DParamMax=[]  NParamMin=[]  NParamMax=[]  KbParamMin=[]  KbParamMax=[]  KtParamMin=[]  KtParamMax=[]  KbOutMin=[]  KbOutMax=[]  KtOutMin=[]  KtOutMax=[]  IntegratorOutMin=[]  IntegratorOutMax=[]  FilterOutMin=[]  FilterOutMax=[]  SumI1OutMin=[]  SumI1OutMax=[]  SumI2OutMin=[]  SumI2OutMax=[]  SumI3OutMin=[]  SumI3OutMax=[]  SumI4OutMin=[]  SumI4OutMax=[]  SumDOutMin=[]  SumDOutMax=[]  DifferentiatorOutMin=[]  DifferentiatorOutMax=[]  FilterDiffOutCoefMin=[]  FilterDiffOutCoefMax=[]  ReciprocalOutMin=[]  ReciprocalOutMax=[]  SumDenOutMin=[]  SumDenOutMax=[]  SumNumOutMin=[]  SumNumOutMax=[]  DivideOutMin=[]  DivideOutMax=[]  UdiffTsProdOutMin=[]  UdiffTsProdOutMax=[]  NTsProdOutMin=[]  NTsProdOutMax=[]  UintegralTsProdOutMin=[]  UintegralTsProdOutMax=[]  UngainTsProdOutMin=[]  UngainTsProdOutMax=[]  ClampingZeroOutDataTypeStr=Inherit: Inherit via back propagation  ClampingZeroOutMin=[]  ClampingZeroOutMax=[]  FilterDenConstantOutDataTypeStr=Inherit: Inherit via back propagation  FilterDenConstantOutMin=[]  FilterDenConstantOutMax=[]  PCopyOutDataTypeStr=Inherit: Inherit via back propagation  PCopyOutMin=[]  PCopyOutMax=[]  NCopyOutDataTypeStr=Inherit: Inherit via back propagation  NCopyOutMin=[]  NCopyOutMax=[]  IntegratorContinuousStateAttributes=''  IntegratorStateMustResolveToSignalObject=off  IntegratorRTWStateStorageClass=Auto  FilterContinuousStateAttributes=''  FilterStateMustResolveToSignalObject=off  FilterRTWStateStorageClass=Auto  ParallelPVariant=InternalParameters  IdealPVariant=Disabled  IVariant=InternalParameters  DVariant=InternalParameters  IntegratorVariant=Continuous  SatVariant=Enabled  AWVariant=BackCalculation  PCopyVariant=Disabled  TRVariant=Disabled  FdbkBlocksVariant=Forward  IdealPFdbkVariant=Disabled  SatFdbkVariant=Disabled  DerivativeFilterVariant=ContFilter  NVariant=InternalParameters  NCopyVariant=Disabled  FilterICVariant=InternalICsFilter  IntegratorICVariant=InternalICs  ExternalResetVariant=Disabled  TRSumVariant=Passthrough  SumFdbkVariant=Disabled  SumVariant=Sum_PID  TsampFilterVariant=InternalTs  TsampNgainVariant=Passthrough  TsampIntegralVariant=Disabled_SignalSpec  ExternalSaturationOutDataTypeStr=Inherit: Same as second input  DerivativeSourceVariant=ErrorSignal  PreIntVariant=InternalPreInt
  Sum2 : Sum  Inputs=|-+
  thetaRef : Outport
  wires:
  Sum2/1 -> PID Controller1/1
  ub/1 -> Sum2/2
  speeduRef/1 -> Sum2/1
  PID Controller1/1 -> thetaRef/1

== system AutogiroModel/Attitude and Altitude Control/Reference Atttiude and Altitude Definition/Lateral Velocity Control ==
  speedvRef : Inport
  vb : Inport  Port=2
  PID Controller1 : slpidlib/PID Controller  Controller=PID  Form=Parallel  TimeDomain=Continuous-time  UseExternalTs=off  SampleTime=-1  IntegratorMethod=Forward Euler  FilterMethod=Forward Euler  ControllerParametersSource=internal  P=0.05  I=0.01  UseKiTs=off  D=0.17  UseExternalDerivativeSource=off  N=100  UseFilter=on  TunerSelectOption=Transfer Function Based (PID Tuner App)  InitialConditionSource=internal  InitialConditionForIntegrator=0  InitialConditionForFilter=0  DifferentiatorICPrevScaledInput=0  ExternalReset=none  TrackingMode=off  Kt=10  LimitOutput=on  SatLimitsSource=internal  UpperSaturationLimit=0.35  LowerSaturationLimit=-0.35  LinearizeAsGain=on  AntiWindupMode=back-calculation  Kb=5  LimitIntegrator=off  UpperIntegratorSaturationLimit=inf  LowerIntegratorSaturationLimit=-inf  POutMin=[]  POutMax=[]  IOutMin=[]  IOutMax=[]  DOutMin=[]  DOutMax=[]  NOutMin=[]  NOutMax=[]  SumOutMin=[]  SumOutMax=[]  SaturationOutMin=[]  SaturationOutMax=[]  PParamMin=[]  PParamMax=[]  IParamMin=[]  IParamMax=[]  DParamMin=[]  DParamMax=[]  NParamMin=[]  NParamMax=[]  KbParamMin=[]  KbParamMax=[]  KtParamMin=[]  KtParamMax=[]  KbOutMin=[]  KbOutMax=[]  KtOutMin=[]  KtOutMax=[]  IntegratorOutMin=[]  IntegratorOutMax=[]  FilterOutMin=[]  FilterOutMax=[]  SumI1OutMin=[]  SumI1OutMax=[]  SumI2OutMin=[]  SumI2OutMax=[]  SumI3OutMin=[]  SumI3OutMax=[]  SumI4OutMin=[]  SumI4OutMax=[]  SumDOutMin=[]  SumDOutMax=[]  DifferentiatorOutMin=[]  DifferentiatorOutMax=[]  FilterDiffOutCoefMin=[]  FilterDiffOutCoefMax=[]  ReciprocalOutMin=[]  ReciprocalOutMax=[]  SumDenOutMin=[]  SumDenOutMax=[]  SumNumOutMin=[]  SumNumOutMax=[]  DivideOutMin=[]  DivideOutMax=[]  UdiffTsProdOutMin=[]  UdiffTsProdOutMax=[]  NTsProdOutMin=[]  NTsProdOutMax=[]  UintegralTsProdOutMin=[]  UintegralTsProdOutMax=[]  UngainTsProdOutMin=[]  UngainTsProdOutMax=[]  ClampingZeroOutDataTypeStr=Inherit: Inherit via back propagation  ClampingZeroOutMin=[]  ClampingZeroOutMax=[]  FilterDenConstantOutDataTypeStr=Inherit: Inherit via back propagation  FilterDenConstantOutMin=[]  FilterDenConstantOutMax=[]  PCopyOutDataTypeStr=Inherit: Inherit via back propagation  PCopyOutMin=[]  PCopyOutMax=[]  NCopyOutDataTypeStr=Inherit: Inherit via back propagation  NCopyOutMin=[]  NCopyOutMax=[]  IntegratorContinuousStateAttributes=''  IntegratorStateMustResolveToSignalObject=off  IntegratorRTWStateStorageClass=Auto  FilterContinuousStateAttributes=''  FilterStateMustResolveToSignalObject=off  FilterRTWStateStorageClass=Auto  ParallelPVariant=InternalParameters  IdealPVariant=Disabled  IVariant=InternalParameters  DVariant=InternalParameters  IntegratorVariant=Continuous  SatVariant=Enabled  AWVariant=BackCalculation  PCopyVariant=Disabled  TRVariant=Disabled  FdbkBlocksVariant=Forward  IdealPFdbkVariant=Disabled  SatFdbkVariant=Disabled  DerivativeFilterVariant=ContFilter  NVariant=InternalParameters  NCopyVariant=Disabled  FilterICVariant=InternalICsFilter  IntegratorICVariant=InternalICs  ExternalResetVariant=Disabled  TRSumVariant=Passthrough  SumFdbkVariant=Disabled  SumVariant=Sum_PID  TsampFilterVariant=InternalTs  TsampNgainVariant=Passthrough  TsampIntegralVariant=Disabled_SignalSpec  ExternalSaturationOutDataTypeStr=Inherit: Same as second input  DerivativeSourceVariant=ErrorSignal  PreIntVariant=InternalPreInt
  Sum2 : Sum  Inputs=|+-
  phiRef : Outport
  wires:
  Sum2/1 -> PID Controller1/1
  PID Controller1/1 -> phiRef/1
  vb/1 -> Sum2/2
  speedvRef/1 -> Sum2/1

== system AutogiroModel/Attitude and Altitude Control/Reference Atttiude and Altitude Definition/Variant Subsystem ==
  note: Set state = "hover" to hover and state = "level" to perform level flight operations
  VRef : Inport
  Vb : Inport  Port=2
  Hover : Subsystem  VariantControl="state == \"hover\""
  Level : Subsystem  VariantControl="state == \"level\" || state == \"path\""
  ub : Outport
